simulink model "CNNLSTM_LHD_states_v1"  (R2019a)
settings: Solver=FixedStepDiscrete  StartTime=0.0  StopTime=2.5  FixedStep=1e-4  RelTol=1e-3
libraries: dspstat3 x1
settings Model: Creator=marceca  LastModifiedBy=marceca

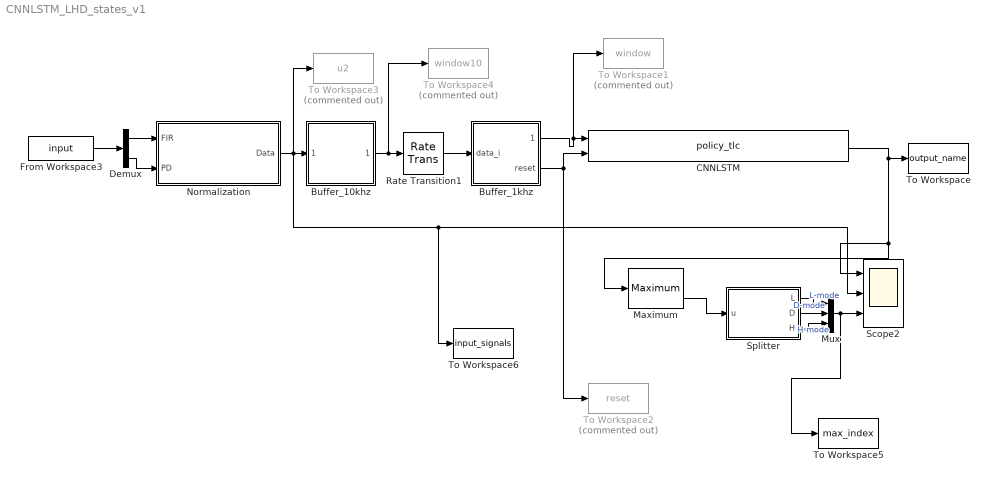
== system CNNLSTM_LHD_states_v1 ==
  Buffer_10khz : Subsystem
  Buffer_1khz : Subsystem
  CNNLSTM : S-Function  FunctionName=policy_tlc  SFunctionDeploymentMode=off  EnableBusSupport=off  mask(Legacy Function){SFunctionSpec=run(single u1[2][40], single y1[3], boolean u2), ShowSpec=on}
      mask prompts: ShowSpec "Display function specification"
      mask help:
      | This block allows you to call the legacy functions specified by the following Legacy Code Tool definition:
      | def.SFunctionName = 'policy_tlc';
      | def.OutputFcnSpec = 'run(single u1[2][40], single y1[3], boolean u2)';
      | def.StartFcnSpec = 'CreateNetwork()';
      | def.TerminateFcnSpec = 'DeleteNetwork()';
      | def.HeaderFiles = {'CNNLSTM_LHD_states.h'};
      | def.HostLibFiles = {'lib_CNNLSTM_LHD_states_03032021.so'};
      | def.TargetLibFiles = {'lib_CNNLSTM_LHD_states_03032021.so'};
      | def.IncPaths = {'inc'};
      | def.LibPaths = {'lib'};
      mask Help: <p>This block was generated automatically by the Legacy Code Tool. For detailed help on this tool, call<a href="matlab:legacy_code('help')"> legacy_code('help')</a>.</p>
      mask Callback ShowSpec:
      | if strcmp(get_param(gcbh, 'ShowSpec'), 'on')
      |   set_param(gcbh, 'MaskDisplay', sprintf('fprintf(''%s'');', get_param(gcbh, 'SFunctionSpec')));
      | else
      |   set_param(gcbh, 'MaskDisplay', sprintf('fprintf(''%s'');', get_param(gcbh, 'FunctionName')));
      | end
      mask Display: fprintf('run(single u1[2][40], single y1[3], boolean u2)');
  Demux : Demux  Outputs=2
  From Workspace3 : FromWorkspace  VariableName=input  SampleTime=0
  Maximum : dspstat3/Maximum  operation=maximum  fcn=Value and Index  indexBase=One  operateOver=Each column  Dimension=1  InputProcessing=Columns as channels (frame based)  reset=None  roiEnable=off  roiType=Rectangles  roiPortion=Entire ROI  roiOutput=Individual statistics for each ROI  roiFlag=off  roundingMode=Floor  overflowMode=off  accumDataTypeStr=Inherit: Same as product output  accumLastDataTypeStr=Inherit: Same as product output
  Mux : Mux  Inputs=3
  Normalization : Subsystem
  Rate Transition1 : RateTransition  OutPortSampleTime=1e-3
  Scope2 : Scope  NumInputPorts=3
  Splitter : MATLAB Function  TreatAsAtomicUnit=on
  To Workspace : ToWorkspace  VariableName=output_name  SaveFormat=Timeseries  SampleTime=-1
  To Workspace1 : ToWorkspace  Commented=on  VariableName=window  SaveFormat=Timeseries  SampleTime=-1
  To Workspace2 : ToWorkspace  Commented=on  VariableName=reset  SaveFormat=Timeseries  SampleTime=-1
  To Workspace3 : ToWorkspace  Commented=on  VariableName=u2  SaveFormat=Timeseries  SampleTime=-1
  To Workspace4 : ToWorkspace  Commented=on  VariableName=window10  SaveFormat=Timeseries  SampleTime=-1
  To Workspace5 : ToWorkspace  VariableName=max_index  SaveFormat=Timeseries  SampleTime=-1
  To Workspace6 : ToWorkspace  VariableName=input_signals  SaveFormat=Timeseries  SampleTime=-1
  wires:
  Demux/1 -> Normalization/1(FIR)
  Demux/2 -> Normalization/2(PD)
  Buffer_10khz/1(window_t_10khz) -> To Workspace4/1, Rate Transition1/1
  Buffer_1khz/1(window_t) -> CNNLSTM/1, To Workspace1/1
  Rate Transition1/1 -> Buffer_1khz/1(data_i)
  CNNLSTM/1 -> Maximum/1, Scope2/1, To Workspace/1
  Buffer_1khz/2(reset) -> CNNLSTM/2, To Workspace2/1
  Normalization/1(Data) -> To Workspace6/1, Scope2/2, Buffer_10khz/1(data_i_10khz), To Workspace3/1
  From Workspace3/1 -> Demux/1
  Maximum/2 -> Splitter/1(u)
  Splitter/1(L) -> Mux/1  "L-mode"
  Splitter/2(D) -> Mux/2  "D-mode"
  Splitter/3(H) -> Mux/3  "H-mode"
  Mux/1 -> To Workspace5/1, Scope2/3

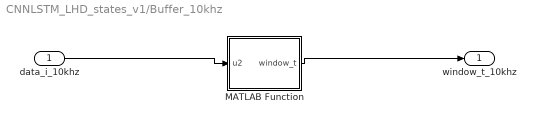
== system CNNLSTM_LHD_states_v1/Buffer_10khz ==
  data_i_10khz : Inport
  MATLAB Function : MATLAB Function  TreatAsAtomicUnit=on
  window_t_10khz : Outport
  wires:
  MATLAB Function/1(window_t) -> window_t_10khz/1
  data_i_10khz/1 -> MATLAB Function/1(u2)

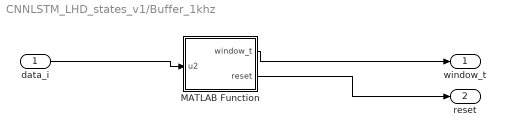
== system CNNLSTM_LHD_states_v1/Buffer_1khz ==
  data_i : Inport
  MATLAB Function : MATLAB Function  TreatAsAtomicUnit=on
  window_t : Outport
  reset : Outport  Port=2
  wires:
  MATLAB Function/1(window_t) -> window_t/1
  data_i/1 -> MATLAB Function/1(u2)
  MATLAB Function/2(reset) -> reset/1

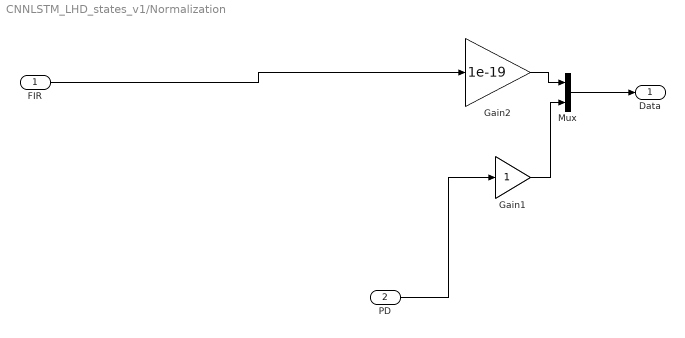
== system CNNLSTM_LHD_states_v1/Normalization ==
  FIR : Inport
  PD : Inport  Port=2
  Gain1 : Gain
  Gain2 : Gain  Gain=1e-19
  Mux : Mux  Inputs=2
  Data : Outport
  wires:
  Gain2/1 -> Mux/1
  Gain1/1 -> Mux/2
  Mux/1 -> Data/1
  FIR/1 -> Gain2/1
  PD/1 -> Gain1/1

== matlab function CNNLSTM_LHD_states_v1/Buffer_10khz/MATLAB Function ==
  data: u2 input; window_t output single
function window_t  = buffer_10khz(u2)
%#codegen
[window_t] =buffer_func_10khz(u2);

== matlab function CNNLSTM_LHD_states_v1/Buffer_1khz/MATLAB Function ==
  data: u2 input; window_t output single; reset output
function [window_t, reset] = buffer_1_khz(u2)
%#codegen
[window_t, reset] = buffer_func_1khz(u2);

== matlab function CNNLSTM_LHD_states_v1/Splitter ==
  data: u input; L output; D output; H output
function [L,D,H]  = splitter(u)

L = u == 1;
D = u == 2;
H = u == 3;
